simulink model "final_version_control_2026_03_26"  (R2024b)
settings: Solver=FixedStepAuto  StartTime=0.0  StopTime=sim  FixedStep=0.01  RelTol=1e-3  EnableMultiTasking=on
undefined symbols (not defined in the file or in its folder): array, Discrete, K, qbreak, Time
libraries: simulink x71, arduinolib x30, dspswit3 x13, arduinosensorlib x2, ctrlSharedLib x2
(part 3 of 4)

== system final_version_control_2026_03_26/Subsystem3/Right Motor Velocity/Subsystem/Subsystem2 ==
  Enable : Inport
  Velocity : Inport  Port=2
  Mux1 : Mux  Inputs=5
  Subsystem : Subsystem
  Subsystem2 : Subsystem
  Enter_motor_mode : Outport
  Velocity_value : Outport  Port=2
  wires:
  Subsystem2/3(Out3) -> Mux1/3
  Subsystem2/2(Out2) -> Mux1/2
  Subsystem2/4(Out4) -> Mux1/4
  Subsystem2/1(Out1) -> Mux1/1
  Subsystem/1(Out1) -> Velocity_value/1
  Mux1/1 -> Enter_motor_mode/1
  Enable/1 -> Mux1/5
  Velocity/1 -> Subsystem/1(In1)

== system final_version_control_2026_03_26/Subsystem1/Left Motor Velocity1/Motor Actual Position Receive/CHINESE CORRECTION/Subsystem ==
  In1 : Inport
  Enable : EnablePort
  Memory : Memory
  Sum : Sum  Inputs=|++
  Out1 : Outport
  wires:
  In1/1 -> Sum/1
  Sum/1 -> Out1/1, Memory/1
  Memory/1 -> Sum/2

== system final_version_control_2026_03_26/Subsystem1/Left Motor Velocity1/Motor Actual Position Receive/Unpack2/Subsystem ==
  In1 : Inport
  In2 : Inport  Port=2
  In3 : Inport  Port=3
  In4 : Inport  Port=4
  In5 : Inport  Port=5
  Bitwise AND : simulink/Logic and Bit Operations/Bitwise Operator  logicop=AND  UseBitMask=on  BitMask=bin2dec('0000000000001111')  BitMaskRealWorld=Stored Integer
  Bitwise OR : simulink/Logic and Bit Operations/Bitwise Operator  logicop=OR  UseBitMask=off  NumInputPorts=2  BitMask=bin2dec('11011001')  BitMaskRealWorld=Stored Integer
  Bitwise OR1 : simulink/Logic and Bit Operations/Bitwise Operator  logicop=OR  UseBitMask=off  NumInputPorts=2  BitMask=bin2dec('11011001')  BitMaskRealWorld=Stored Integer
  Bitwise OR2 : simulink/Logic and Bit Operations/Bitwise Operator  logicop=OR  UseBitMask=off  NumInputPorts=2  BitMask=bin2dec('11011001')  BitMaskRealWorld=Stored Integer
  Constant : Constant  Value=8  OutDataTypeStr=uint16
  Constant1 : Constant  Value=4  OutDataTypeStr=uint16
  Constant2 : Constant  Value=4  OutDataTypeStr=uint16
  Constant4 : Constant  Value=8  OutDataTypeStr=uint16
  Shift Arithmetic1 : ArithShift  BitShiftNumberSource=Input port  BitShiftNumber=8  BitShiftDirection=Left
  Shift Arithmetic2 : ArithShift  BitShiftNumberSource=Input port  BitShiftNumber=8  BitShiftDirection=Left
  Shift Arithmetic3 : ArithShift  BitShiftNumberSource=Input port  BitShiftNumber=8  BitShiftDirection=Right
  Shift Arithmetic4 : ArithShift  BitShiftNumberSource=Input port  BitShiftNumber=8  BitShiftDirection=Left
  Out1 : Outport
  Out2 : Outport  Port=2
  Out3 : Outport  Port=3
  wires:
  Bitwise AND/1 -> Shift Arithmetic4/1
  In5/1 -> Bitwise OR2/1
  Shift Arithmetic1/1 -> Bitwise OR1/1
  In1/1 -> Shift Arithmetic1/1
  Shift Arithmetic2/1 -> Bitwise OR/1
  Shift Arithmetic3/1 -> Bitwise OR/2
  Shift Arithmetic4/1 -> Bitwise OR2/2
  In2/1 -> Bitwise OR1/2
  Bitwise OR1/1 -> Out1/1
  Bitwise OR2/1 -> Out3/1
  In3/1 -> Shift Arithmetic2/1
  Constant4/1 -> Shift Arithmetic4/2
  Constant2/1 -> Shift Arithmetic3/2
  Constant1/1 -> Shift Arithmetic2/2
  Constant/1 -> Shift Arithmetic1/2
  Bitwise OR/1 -> Out2/1
  In4/1 -> Shift Arithmetic3/1, Bitwise AND/1

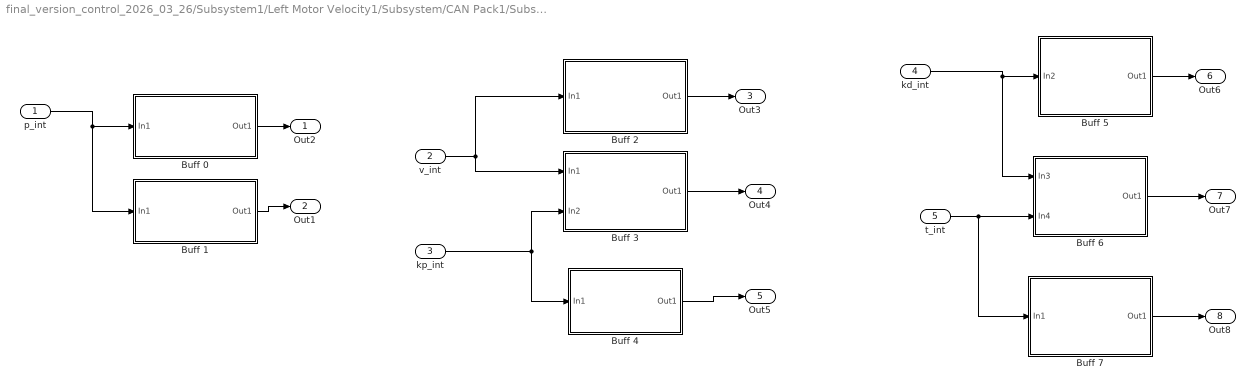
== system final_version_control_2026_03_26/Subsystem1/Left Motor Velocity1/Subsystem/CAN Pack1/Subsystem ==
  p_int : Inport
  v_int : Inport  Port=2
  kp_int : Inport  Port=3
  kd_int : Inport  Port=4
  t_int : Inport  Port=5
  Buff 0 : Subsystem
  Buff 1 : Subsystem
  Buff 2 : Subsystem
  Buff 3 : Subsystem
  Buff 4 : Subsystem
  Buff 5 : Subsystem
  Buff 6 : Subsystem
  Buff 7 : Subsystem
  Out2 : Outport
  Out1 : Outport  Port=2
  Out3 : Outport  Port=3
  Out4 : Outport  Port=4
  Out5 : Outport  Port=5
  Out6 : Outport  Port=6
  Out7 : Outport  Port=7
  Out8 : Outport  Port=8
  wires:
  Buff 5/1(Out1) -> Out6/1
  Buff 7/1(Out1) -> Out8/1
  Buff 6/1(Out1) -> Out7/1
  Buff 0/1(Out1) -> Out2/1
  Buff 1/1(Out1) -> Out1/1
  Buff 2/1(Out1) -> Out3/1
  Buff 4/1(Out1) -> Out5/1
  Buff 3/1(Out1) -> Out4/1
  p_int/1 -> Buff 0/1(In1), Buff 1/1(In1)
  v_int/1 -> Buff 3/1(In1), Buff 2/1(In1)
  kd_int/1 -> Buff 6/1(In3), Buff 5/1(In2)
  kp_int/1 -> Buff 3/2(In2), Buff 4/1(In1)
  t_int/1 -> Buff 7/1(In1), Buff 6/2(In4)

== system final_version_control_2026_03_26/Subsystem1/Left Motor Velocity1/Subsystem/Subsystem2/Subsystem ==
  In1 : Inport
  Kd : Constant  OutDataTypeStr=single
  Kp : Constant  Value=0  OutDataTypeStr=single
  Mux2 : Mux  Inputs=5
  Position Command : Constant  Value=0  VectorParams1D=off  OutDataTypeStr=single
  Saturation : Saturate  UpperLimit=12.5  LowerLimit=-12.5
  Saturation1 : Saturate  UpperLimit=41.87  LowerLimit=-41.87
  Saturation2 : Saturate  UpperLimit=500  LowerLimit=0
  Saturation3 : Saturate  UpperLimit=5  LowerLimit=0
  Saturation4 : Saturate  UpperLimit=9  LowerLimit=-9
  Torque : Constant  Value=0  OutDataTypeStr=single
  Out1 : Outport
  wires:
  Saturation/1 -> Mux2/1
  Kp/1 -> Saturation2/1
  In1/1 -> Saturation1/1
  Position Command/1 -> Saturation/1
  Saturation1/1 -> Mux2/2
  Kd/1 -> Saturation3/1
  Saturation4/1 -> Mux2/5
  Torque/1 -> Saturation4/1
  Saturation2/1 -> Mux2/3
  Saturation3/1 -> Mux2/4
  Mux2/1 -> Out1/1

== system final_version_control_2026_03_26/Subsystem1/Left Motor Velocity1/Subsystem/Subsystem2/Subsystem2 ==
  Kd1 : Constant  Value=5  OutDataTypeStr=single
  Kp1 : Constant  Value=500  OutDataTypeStr=single
  Position Command1 : Constant  Value=12.5  VectorParams1D=off  OutDataTypeStr=single
  Velocity Command1 : Constant  Value=45  OutDataTypeStr=single
  Out1 : Outport
  Out2 : Outport  Port=2
  Out3 : Outport  Port=3
  Out4 : Outport  Port=4
  wires:
  Kd1/1 -> Out4/1
  Position Command1/1 -> Out1/1
  Velocity Command1/1 -> Out2/1
  Kp1/1 -> Out3/1

== system final_version_control_2026_03_26/Subsystem1/Right Motor Velocity1/Motor Actual Position Receive/CHINESE CORRECTION/Subsystem ==
  In1 : Inport
  Enable : EnablePort
  Memory : Memory
  Sum : Sum  Inputs=|++
  Out1 : Outport
  wires:
  In1/1 -> Sum/1
  Sum/1 -> Out1/1, Memory/1
  Memory/1 -> Sum/2

== system final_version_control_2026_03_26/Subsystem1/Right Motor Velocity1/Motor Actual Position Receive/Unpack2/Subsystem ==
  In1 : Inport
  In2 : Inport  Port=2
  In3 : Inport  Port=3
  In4 : Inport  Port=4
  In5 : Inport  Port=5
  Bitwise AND : simulink/Logic and Bit Operations/Bitwise Operator  logicop=AND  UseBitMask=on  BitMask=bin2dec('0000000000001111')  BitMaskRealWorld=Stored Integer
  Bitwise OR : simulink/Logic and Bit Operations/Bitwise Operator  logicop=OR  UseBitMask=off  NumInputPorts=2  BitMask=bin2dec('11011001')  BitMaskRealWorld=Stored Integer
  Bitwise OR1 : simulink/Logic and Bit Operations/Bitwise Operator  logicop=OR  UseBitMask=off  NumInputPorts=2  BitMask=bin2dec('11011001')  BitMaskRealWorld=Stored Integer
  Bitwise OR2 : simulink/Logic and Bit Operations/Bitwise Operator  logicop=OR  UseBitMask=off  NumInputPorts=2  BitMask=bin2dec('11011001')  BitMaskRealWorld=Stored Integer
  Constant : Constant  Value=8  OutDataTypeStr=uint16
  Constant1 : Constant  Value=4  OutDataTypeStr=uint16
  Constant2 : Constant  Value=4  OutDataTypeStr=uint16
  Constant4 : Constant  Value=8  OutDataTypeStr=uint16
  Shift Arithmetic1 : ArithShift  BitShiftNumberSource=Input port  BitShiftNumber=8  BitShiftDirection=Left
  Shift Arithmetic2 : ArithShift  BitShiftNumberSource=Input port  BitShiftNumber=8  BitShiftDirection=Left
  Shift Arithmetic3 : ArithShift  BitShiftNumberSource=Input port  BitShiftNumber=8  BitShiftDirection=Right
  Shift Arithmetic4 : ArithShift  BitShiftNumberSource=Input port  BitShiftNumber=8  BitShiftDirection=Left
  Out1 : Outport
  Out2 : Outport  Port=2
  Out3 : Outport  Port=3
  wires:
  Bitwise AND/1 -> Shift Arithmetic4/1
  In5/1 -> Bitwise OR2/1
  Shift Arithmetic1/1 -> Bitwise OR1/1
  In1/1 -> Shift Arithmetic1/1
  Shift Arithmetic2/1 -> Bitwise OR/1
  Shift Arithmetic3/1 -> Bitwise OR/2
  Shift Arithmetic4/1 -> Bitwise OR2/2
  In2/1 -> Bitwise OR1/2
  Bitwise OR1/1 -> Out1/1
  Bitwise OR2/1 -> Out3/1
  In3/1 -> Shift Arithmetic2/1
  Constant4/1 -> Shift Arithmetic4/2
  Constant2/1 -> Shift Arithmetic3/2
  Constant1/1 -> Shift Arithmetic2/2
  Constant/1 -> Shift Arithmetic1/2
  Bitwise OR/1 -> Out2/1
  In4/1 -> Shift Arithmetic3/1, Bitwise AND/1

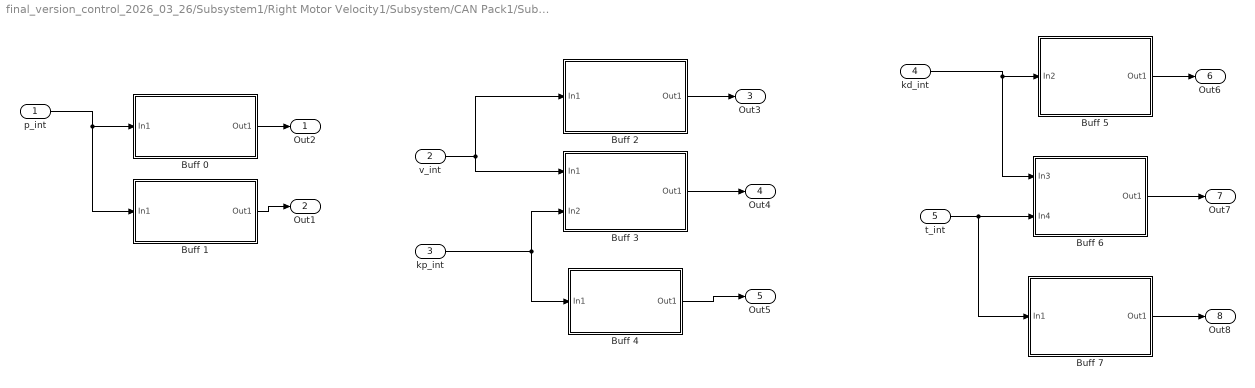
== system final_version_control_2026_03_26/Subsystem1/Right Motor Velocity1/Subsystem/CAN Pack1/Subsystem ==
  p_int : Inport
  v_int : Inport  Port=2
  kp_int : Inport  Port=3
  kd_int : Inport  Port=4
  t_int : Inport  Port=5
  Buff 0 : Subsystem
  Buff 1 : Subsystem
  Buff 2 : Subsystem
  Buff 3 : Subsystem
  Buff 4 : Subsystem
  Buff 5 : Subsystem
  Buff 6 : Subsystem
  Buff 7 : Subsystem
  Out2 : Outport
  Out1 : Outport  Port=2
  Out3 : Outport  Port=3
  Out4 : Outport  Port=4
  Out5 : Outport  Port=5
  Out6 : Outport  Port=6
  Out7 : Outport  Port=7
  Out8 : Outport  Port=8
  wires:
  Buff 5/1(Out1) -> Out6/1
  Buff 7/1(Out1) -> Out8/1
  Buff 6/1(Out1) -> Out7/1
  Buff 0/1(Out1) -> Out2/1
  Buff 1/1(Out1) -> Out1/1
  Buff 2/1(Out1) -> Out3/1
  Buff 4/1(Out1) -> Out5/1
  Buff 3/1(Out1) -> Out4/1
  p_int/1 -> Buff 0/1(In1), Buff 1/1(In1)
  v_int/1 -> Buff 3/1(In1), Buff 2/1(In1)
  kd_int/1 -> Buff 6/1(In3), Buff 5/1(In2)
  kp_int/1 -> Buff 3/2(In2), Buff 4/1(In1)
  t_int/1 -> Buff 7/1(In1), Buff 6/2(In4)

== system final_version_control_2026_03_26/Subsystem1/Right Motor Velocity1/Subsystem/Subsystem2/Subsystem ==
  In1 : Inport
  Kd : Constant  OutDataTypeStr=single
  Kp : Constant  Value=0  OutDataTypeStr=single
  Mux2 : Mux  Inputs=5
  Position Command : Constant  Value=0  VectorParams1D=off  OutDataTypeStr=single
  Saturation : Saturate  UpperLimit=12.5  LowerLimit=-12.5
  Saturation1 : Saturate  UpperLimit=41.87  LowerLimit=-41.87
  Saturation2 : Saturate  UpperLimit=500  LowerLimit=0
  Saturation3 : Saturate  UpperLimit=5  LowerLimit=0
  Saturation4 : Saturate  UpperLimit=9  LowerLimit=-9
  Torque : Constant  Value=0  OutDataTypeStr=single
  Out1 : Outport
  wires:
  Saturation/1 -> Mux2/1
  Kp/1 -> Saturation2/1
  In1/1 -> Saturation1/1
  Position Command/1 -> Saturation/1
  Saturation1/1 -> Mux2/2
  Kd/1 -> Saturation3/1
  Saturation4/1 -> Mux2/5
  Torque/1 -> Saturation4/1
  Saturation2/1 -> Mux2/3
  Saturation3/1 -> Mux2/4
  Mux2/1 -> Out1/1

== system final_version_control_2026_03_26/Subsystem1/Right Motor Velocity1/Subsystem/Subsystem2/Subsystem2 ==
  Kd1 : Constant  Value=5  OutDataTypeStr=single
  Kp1 : Constant  Value=500  OutDataTypeStr=single
  Position Command1 : Constant  Value=12.5  VectorParams1D=off  OutDataTypeStr=single
  Velocity Command1 : Constant  Value=45  OutDataTypeStr=single
  Out1 : Outport
  Out2 : Outport  Port=2
  Out3 : Outport  Port=3
  Out4 : Outport  Port=4
  wires:
  Kd1/1 -> Out4/1
  Position Command1/1 -> Out1/1
  Velocity Command1/1 -> Out2/1
  Kp1/1 -> Out3/1

== system final_version_control_2026_03_26/Subsystem3/Left Motor Velocity/Motor Actual Position Receive/CHINESE CORRECTION/Subsystem ==
  In1 : Inport
  Enable : EnablePort
  Memory : Memory
  Sum : Sum  Inputs=|++
  Out1 : Outport
  wires:
  In1/1 -> Sum/1
  Sum/1 -> Out1/1, Memory/1
  Memory/1 -> Sum/2

== system final_version_control_2026_03_26/Subsystem3/Left Motor Velocity/Motor Actual Position Receive/Unpack2/Subsystem ==
  In1 : Inport
  In2 : Inport  Port=2
  In3 : Inport  Port=3
  In4 : Inport  Port=4
  In5 : Inport  Port=5
  Bitwise AND : simulink/Logic and Bit Operations/Bitwise Operator  logicop=AND  UseBitMask=on  BitMask=bin2dec('0000000000001111')  BitMaskRealWorld=Stored Integer
  Bitwise OR : simulink/Logic and Bit Operations/Bitwise Operator  logicop=OR  UseBitMask=off  NumInputPorts=2  BitMask=bin2dec('11011001')  BitMaskRealWorld=Stored Integer
  Bitwise OR1 : simulink/Logic and Bit Operations/Bitwise Operator  logicop=OR  UseBitMask=off  NumInputPorts=2  BitMask=bin2dec('11011001')  BitMaskRealWorld=Stored Integer
  Bitwise OR2 : simulink/Logic and Bit Operations/Bitwise Operator  logicop=OR  UseBitMask=off  NumInputPorts=2  BitMask=bin2dec('11011001')  BitMaskRealWorld=Stored Integer
  Constant : Constant  Value=8  OutDataTypeStr=uint16
  Constant1 : Constant  Value=4  OutDataTypeStr=uint16
  Constant2 : Constant  Value=4  OutDataTypeStr=uint16
  Constant4 : Constant  Value=8  OutDataTypeStr=uint16
  Shift Arithmetic1 : ArithShift  BitShiftNumberSource=Input port  BitShiftNumber=8  BitShiftDirection=Left
  Shift Arithmetic2 : ArithShift  BitShiftNumberSource=Input port  BitShiftNumber=8  BitShiftDirection=Left
  Shift Arithmetic3 : ArithShift  BitShiftNumberSource=Input port  BitShiftNumber=8  BitShiftDirection=Right
  Shift Arithmetic4 : ArithShift  BitShiftNumberSource=Input port  BitShiftNumber=8  BitShiftDirection=Left
  Out1 : Outport
  Out2 : Outport  Port=2
  Out3 : Outport  Port=3
  wires:
  Bitwise AND/1 -> Shift Arithmetic4/1
  In5/1 -> Bitwise OR2/1
  Shift Arithmetic1/1 -> Bitwise OR1/1
  In1/1 -> Shift Arithmetic1/1
  Shift Arithmetic2/1 -> Bitwise OR/1
  Shift Arithmetic3/1 -> Bitwise OR/2
  Shift Arithmetic4/1 -> Bitwise OR2/2
  In2/1 -> Bitwise OR1/2
  Bitwise OR1/1 -> Out1/1
  Bitwise OR2/1 -> Out3/1
  In3/1 -> Shift Arithmetic2/1
  Constant4/1 -> Shift Arithmetic4/2
  Constant2/1 -> Shift Arithmetic3/2
  Constant1/1 -> Shift Arithmetic2/2
  Constant/1 -> Shift Arithmetic1/2
  Bitwise OR/1 -> Out2/1
  In4/1 -> Shift Arithmetic3/1, Bitwise AND/1

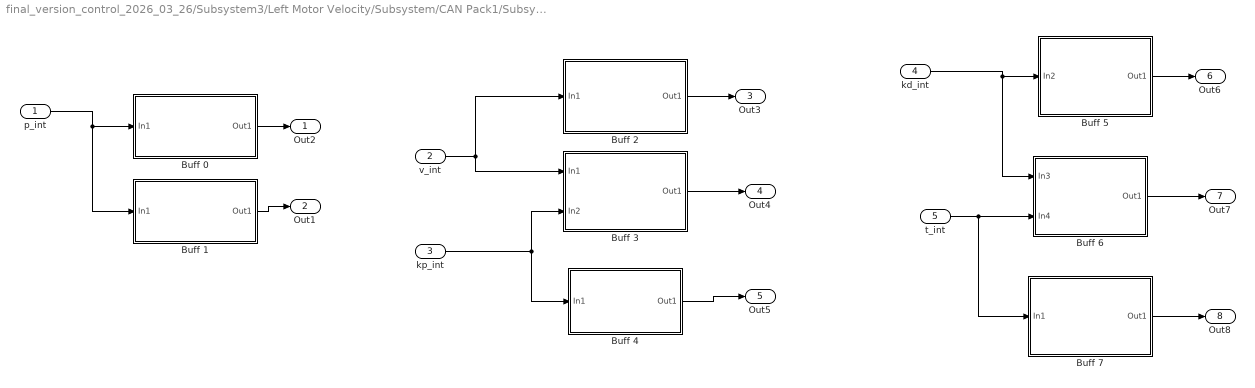
== system final_version_control_2026_03_26/Subsystem3/Left Motor Velocity/Subsystem/CAN Pack1/Subsystem ==
  p_int : Inport
  v_int : Inport  Port=2
  kp_int : Inport  Port=3
  kd_int : Inport  Port=4
  t_int : Inport  Port=5
  Buff 0 : Subsystem
  Buff 1 : Subsystem
  Buff 2 : Subsystem
  Buff 3 : Subsystem
  Buff 4 : Subsystem
  Buff 5 : Subsystem
  Buff 6 : Subsystem
  Buff 7 : Subsystem
  Out2 : Outport
  Out1 : Outport  Port=2
  Out3 : Outport  Port=3
  Out4 : Outport  Port=4
  Out5 : Outport  Port=5
  Out6 : Outport  Port=6
  Out7 : Outport  Port=7
  Out8 : Outport  Port=8
  wires:
  Buff 5/1(Out1) -> Out6/1
  Buff 7/1(Out1) -> Out8/1
  Buff 6/1(Out1) -> Out7/1
  Buff 0/1(Out1) -> Out2/1
  Buff 1/1(Out1) -> Out1/1
  Buff 2/1(Out1) -> Out3/1
  Buff 4/1(Out1) -> Out5/1
  Buff 3/1(Out1) -> Out4/1
  p_int/1 -> Buff 0/1(In1), Buff 1/1(In1)
  v_int/1 -> Buff 3/1(In1), Buff 2/1(In1)
  kd_int/1 -> Buff 6/1(In3), Buff 5/1(In2)
  kp_int/1 -> Buff 3/2(In2), Buff 4/1(In1)
  t_int/1 -> Buff 7/1(In1), Buff 6/2(In4)

== system final_version_control_2026_03_26/Subsystem3/Left Motor Velocity/Subsystem/Subsystem2/Subsystem ==
  In1 : Inport
  Kd : Constant  OutDataTypeStr=single
  Kp : Constant  Value=0  OutDataTypeStr=single
  Mux2 : Mux  Inputs=5
  Position Command : Constant  Value=0  VectorParams1D=off  OutDataTypeStr=single
  Saturation : Saturate  UpperLimit=12.5  LowerLimit=-12.5
  Saturation1 : Saturate  UpperLimit=41.87  LowerLimit=-41.87
  Saturation2 : Saturate  UpperLimit=500  LowerLimit=0
  Saturation3 : Saturate  UpperLimit=5  LowerLimit=0
  Saturation4 : Saturate  UpperLimit=9  LowerLimit=-9
  Torque : Constant  Value=0  OutDataTypeStr=single
  Out1 : Outport
  wires:
  Saturation/1 -> Mux2/1
  Kp/1 -> Saturation2/1
  In1/1 -> Saturation1/1
  Position Command/1 -> Saturation/1
  Saturation1/1 -> Mux2/2
  Kd/1 -> Saturation3/1
  Saturation4/1 -> Mux2/5
  Torque/1 -> Saturation4/1
  Saturation2/1 -> Mux2/3
  Saturation3/1 -> Mux2/4
  Mux2/1 -> Out1/1

== system final_version_control_2026_03_26/Subsystem3/Left Motor Velocity/Subsystem/Subsystem2/Subsystem2 ==
  Kd1 : Constant  Value=5  OutDataTypeStr=single
  Kp1 : Constant  Value=500  OutDataTypeStr=single
  Position Command1 : Constant  Value=12.5  VectorParams1D=off  OutDataTypeStr=single
  Velocity Command1 : Constant  Value=45  OutDataTypeStr=single
  Out1 : Outport
  Out2 : Outport  Port=2
  Out3 : Outport  Port=3
  Out4 : Outport  Port=4
  wires:
  Kd1/1 -> Out4/1
  Position Command1/1 -> Out1/1
  Velocity Command1/1 -> Out2/1
  Kp1/1 -> Out3/1

== system final_version_control_2026_03_26/Subsystem3/Right Motor Velocity/Motor Actual Position Receive/CHINESE CORRECTION/Subsystem ==
  In1 : Inport
  Enable : EnablePort
  Memory : Memory
  Sum : Sum  Inputs=|++
  Out1 : Outport
  wires:
  In1/1 -> Sum/1
  Sum/1 -> Out1/1, Memory/1
  Memory/1 -> Sum/2

== system final_version_control_2026_03_26/Subsystem3/Right Motor Velocity/Motor Actual Position Receive/Unpack2/Subsystem ==
  In1 : Inport
  In2 : Inport  Port=2
  In3 : Inport  Port=3
  In4 : Inport  Port=4
  In5 : Inport  Port=5
  Bitwise AND : simulink/Logic and Bit Operations/Bitwise Operator  logicop=AND  UseBitMask=on  BitMask=bin2dec('0000000000001111')  BitMaskRealWorld=Stored Integer
  Bitwise OR : simulink/Logic and Bit Operations/Bitwise Operator  logicop=OR  UseBitMask=off  NumInputPorts=2  BitMask=bin2dec('11011001')  BitMaskRealWorld=Stored Integer
  Bitwise OR1 : simulink/Logic and Bit Operations/Bitwise Operator  logicop=OR  UseBitMask=off  NumInputPorts=2  BitMask=bin2dec('11011001')  BitMaskRealWorld=Stored Integer
  Bitwise OR2 : simulink/Logic and Bit Operations/Bitwise Operator  logicop=OR  UseBitMask=off  NumInputPorts=2  BitMask=bin2dec('11011001')  BitMaskRealWorld=Stored Integer
  Constant : Constant  Value=8  OutDataTypeStr=uint16
  Constant1 : Constant  Value=4  OutDataTypeStr=uint16
  Constant2 : Constant  Value=4  OutDataTypeStr=uint16
  Constant4 : Constant  Value=8  OutDataTypeStr=uint16
  Shift Arithmetic1 : ArithShift  BitShiftNumberSource=Input port  BitShiftNumber=8  BitShiftDirection=Left
  Shift Arithmetic2 : ArithShift  BitShiftNumberSource=Input port  BitShiftNumber=8  BitShiftDirection=Left
  Shift Arithmetic3 : ArithShift  BitShiftNumberSource=Input port  BitShiftNumber=8  BitShiftDirection=Right
  Shift Arithmetic4 : ArithShift  BitShiftNumberSource=Input port  BitShiftNumber=8  BitShiftDirection=Left
  Out1 : Outport
  Out2 : Outport  Port=2
  Out3 : Outport  Port=3
  wires:
  Bitwise AND/1 -> Shift Arithmetic4/1
  In5/1 -> Bitwise OR2/1
  Shift Arithmetic1/1 -> Bitwise OR1/1
  In1/1 -> Shift Arithmetic1/1
  Shift Arithmetic2/1 -> Bitwise OR/1
  Shift Arithmetic3/1 -> Bitwise OR/2
  Shift Arithmetic4/1 -> Bitwise OR2/2
  In2/1 -> Bitwise OR1/2
  Bitwise OR1/1 -> Out1/1
  Bitwise OR2/1 -> Out3/1
  In3/1 -> Shift Arithmetic2/1
  Constant4/1 -> Shift Arithmetic4/2
  Constant2/1 -> Shift Arithmetic3/2
  Constant1/1 -> Shift Arithmetic2/2
  Constant/1 -> Shift Arithmetic1/2
  Bitwise OR/1 -> Out2/1
  In4/1 -> Shift Arithmetic3/1, Bitwise AND/1

== system final_version_control_2026_03_26/Subsystem3/Right Motor Velocity/Subsystem/CAN Pack1/Subsystem ==
  p_int : Inport
  v_int : Inport  Port=2
  kp_int : Inport  Port=3
  kd_int : Inport  Port=4
  t_int : Inport  Port=5
  Buff 0 : Subsystem
  Buff 1 : Subsystem
  Buff 2 : Subsystem
  Buff 3 : Subsystem
  Buff 4 : Subsystem
  Buff 5 : Subsystem
  Buff 6 : Subsystem
  Buff 7 : Subsystem
  Out2 : Outport
  Out1 : Outport  Port=2
  Out3 : Outport  Port=3
  Out4 : Outport  Port=4
  Out5 : Outport  Port=5
  Out6 : Outport  Port=6
  Out7 : Outport  Port=7
  Out8 : Outport  Port=8
  wires:
  Buff 5/1(Out1) -> Out6/1
  Buff 7/1(Out1) -> Out8/1
  Buff 6/1(Out1) -> Out7/1
  Buff 0/1(Out1) -> Out2/1
  Buff 1/1(Out1) -> Out1/1
  Buff 2/1(Out1) -> Out3/1
  Buff 4/1(Out1) -> Out5/1
  Buff 3/1(Out1) -> Out4/1
  p_int/1 -> Buff 0/1(In1), Buff 1/1(In1)
  v_int/1 -> Buff 3/1(In1), Buff 2/1(In1)
  kd_int/1 -> Buff 6/1(In3), Buff 5/1(In2)
  kp_int/1 -> Buff 3/2(In2), Buff 4/1(In1)
  t_int/1 -> Buff 7/1(In1), Buff 6/2(In4)

== system final_version_control_2026_03_26/Subsystem3/Right Motor Velocity/Subsystem/Subsystem2/Subsystem ==
  In1 : Inport
  Kd : Constant  OutDataTypeStr=single
  Kp : Constant  Value=0  OutDataTypeStr=single
  Mux2 : Mux  Inputs=5
  Position Command : Constant  Value=0  VectorParams1D=off  OutDataTypeStr=single
  Saturation : Saturate  UpperLimit=12.5  LowerLimit=-12.5
  Saturation1 : Saturate  UpperLimit=41.87  LowerLimit=-41.87
  Saturation2 : Saturate  UpperLimit=500  LowerLimit=0
  Saturation3 : Saturate  UpperLimit=5  LowerLimit=0
  Saturation4 : Saturate  UpperLimit=9  LowerLimit=-9
  Torque : Constant  Value=0  OutDataTypeStr=single
  Out1 : Outport
  wires:
  Saturation/1 -> Mux2/1
  Kp/1 -> Saturation2/1
  In1/1 -> Saturation1/1
  Position Command/1 -> Saturation/1
  Saturation1/1 -> Mux2/2
  Kd/1 -> Saturation3/1
  Saturation4/1 -> Mux2/5
  Torque/1 -> Saturation4/1
  Saturation2/1 -> Mux2/3
  Saturation3/1 -> Mux2/4
  Mux2/1 -> Out1/1

== system final_version_control_2026_03_26/Subsystem3/Right Motor Velocity/Subsystem/Subsystem2/Subsystem2 ==
  Kd1 : Constant  Value=5  OutDataTypeStr=single
  Kp1 : Constant  Value=500  OutDataTypeStr=single
  Position Command1 : Constant  Value=12.5  VectorParams1D=off  OutDataTypeStr=single
  Velocity Command1 : Constant  Value=45  OutDataTypeStr=single
  Out1 : Outport
  Out2 : Outport  Port=2
  Out3 : Outport  Port=3
  Out4 : Outport  Port=4
  wires:
  Kd1/1 -> Out4/1
  Position Command1/1 -> Out1/1
  Velocity Command1/1 -> Out2/1
  Kp1/1 -> Out3/1

== system final_version_control_2026_03_26/Subsystem1/Left Motor Velocity1/Subsystem/CAN Pack1/Subsystem/Buff 0 ==
  In1 : Inport
  Constant1 : Constant  Value=8  OutDataTypeStr=uint16
  Data Type Conversion : DataTypeConversion  OutDataTypeStr=uint8  SaturateOnIntegerOverflow=off  RndMeth=Floor
  Shift Arithmetic2 : ArithShift  BitShiftNumberSource=Input port  BitShiftNumber=8  BitShiftDirection=Right
  Out1 : Outport
  wires:
  In1/1 -> Shift Arithmetic2/1
  Shift Arithmetic2/1 -> Data Type Conversion/1
  Data Type Conversion/1 -> Out1/1
  Constant1/1 -> Shift Arithmetic2/2

== system final_version_control_2026_03_26/Subsystem1/Left Motor Velocity1/Subsystem/CAN Pack1/Subsystem/Buff 1 ==
  In1 : Inport
  Bitwise AND : simulink/Logic and Bit Operations/Bitwise Operator  logicop=AND  UseBitMask=on  BitMask=bin2dec('0000000011111111')  BitMaskRealWorld=Stored Integer
  Data Type Conversion1 : DataTypeConversion  OutDataTypeStr=uint8  SaturateOnIntegerOverflow=off  RndMeth=Floor
  Out1 : Outport
  wires:
  Bitwise AND/1 -> Data Type Conversion1/1
  Data Type Conversion1/1 -> Out1/1
  In1/1 -> Bitwise AND/1

== system final_version_control_2026_03_26/Subsystem1/Left Motor Velocity1/Subsystem/CAN Pack1/Subsystem/Buff 2 ==
  In1 : Inport
  Constant2 : Constant  Value=4  OutDataTypeStr=uint16
  Data Type Conversion2 : DataTypeConversion  OutDataTypeStr=uint8  SaturateOnIntegerOverflow=off  RndMeth=Floor
  Shift Arithmetic1 : ArithShift  BitShiftNumberSource=Input port  BitShiftNumber=8  BitShiftDirection=Right
  Out1 : Outport
  wires:
  Shift Arithmetic1/1 -> Data Type Conversion2/1
  Data Type Conversion2/1 -> Out1/1
  In1/1 -> Shift Arithmetic1/1
  Constant2/1 -> Shift Arithmetic1/2

== system final_version_control_2026_03_26/Subsystem1/Left Motor Velocity1/Subsystem/CAN Pack1/Subsystem/Buff 3 ==
  In1 : Inport
  In2 : Inport  Port=2
  Bitwise AND1 : simulink/Logic and Bit Operations/Bitwise Operator  logicop=AND  UseBitMask=on  BitMask=bin2dec('000000001111')  BitMaskRealWorld=Stored Integer
  Bitwise OR1 : simulink/Logic and Bit Operations/Bitwise Operator  logicop=OR  UseBitMask=off  NumInputPorts=2  BitMask=bin2dec('11011001')  BitMaskRealWorld=Stored Integer
  Constant1 : Constant  Value=8  OutDataTypeStr=uint16
  Constant2 : Constant  Value=4  OutDataTypeStr=uint16
  Data Type Conversion3 : DataTypeConversion  OutDataTypeStr=uint8  SaturateOnIntegerOverflow=off  RndMeth=Floor
  Shift Arithmetic3 : ArithShift  BitShiftNumberSource=Input port  BitShiftNumber=8  BitShiftDirection=Left
  Shift Arithmetic4 : ArithShift  BitShiftNumberSource=Input port  BitShiftNumber=8  BitShiftDirection=Right
  Out1 : Outport
  wires:
  Shift Arithmetic3/1 -> Bitwise OR1/1
  In1/1 -> Bitwise AND1/1
  Constant1/1 -> Shift Arithmetic4/2
  Bitwise AND1/1 -> Shift Arithmetic3/1
  Shift Arithmetic4/1 -> Bitwise OR1/2
  In2/1 -> Shift Arithmetic4/1
  Bitwise OR1/1 -> Data Type Conversion3/1
  Data Type Conversion3/1 -> Out1/1
  Constant2/1 -> Shift Arithmetic3/2

== system final_version_control_2026_03_26/Subsystem1/Left Motor Velocity1/Subsystem/CAN Pack1/Subsystem/Buff 4 ==
  In1 : Inport
  Bitwise AND3 : simulink/Logic and Bit Operations/Bitwise Operator  logicop=AND  UseBitMask=on  BitMask=bin2dec('000011111111')  BitMaskRealWorld=Stored Integer
  Data Type Conversion4 : DataTypeConversion  OutDataTypeStr=uint8  SaturateOnIntegerOverflow=off  RndMeth=Floor
  Out1 : Outport
  wires:
  Data Type Conversion4/1 -> Out1/1
  Bitwise AND3/1 -> Data Type Conversion4/1
  In1/1 -> Bitwise AND3/1

== system final_version_control_2026_03_26/Subsystem1/Left Motor Velocity1/Subsystem/CAN Pack1/Subsystem/Buff 5 ==
  In2 : Inport
  Constant2 : Constant  Value=4  OutDataTypeStr=uint16
  Data Type Conversion5 : DataTypeConversion  OutDataTypeStr=uint8  SaturateOnIntegerOverflow=off  RndMeth=Floor
  Shift Arithmetic5 : ArithShift  BitShiftNumberSource=Input port  BitShiftNumber=8  BitShiftDirection=Right
  Out1 : Outport
  wires:
  In2/1 -> Shift Arithmetic5/1
  Shift Arithmetic5/1 -> Data Type Conversion5/1
  Data Type Conversion5/1 -> Out1/1
  Constant2/1 -> Shift Arithmetic5/2

== system final_version_control_2026_03_26/Subsystem1/Left Motor Velocity1/Subsystem/CAN Pack1/Subsystem/Buff 6 ==
  In3 : Inport
  In4 : Inport  Port=2
  Bitwise AND2 : simulink/Logic and Bit Operations/Bitwise Operator  logicop=AND  UseBitMask=on  BitMask=bin2dec('000000001111')  BitMaskRealWorld=Stored Integer
  Bitwise OR2 : simulink/Logic and Bit Operations/Bitwise Operator  logicop=OR  UseBitMask=off  NumInputPorts=2  BitMask=bin2dec('11011001')  BitMaskRealWorld=Stored Integer
  Constant1 : Constant  Value=8  OutDataTypeStr=uint16
  Constant2 : Constant  Value=4  OutDataTypeStr=uint16
  Data Type Conversion6 : DataTypeConversion  OutDataTypeStr=uint8  SaturateOnIntegerOverflow=off  RndMeth=Floor
  Shift Arithmetic6 : ArithShift  BitShiftNumberSource=Input port  BitShiftNumber=8  BitShiftDirection=Left
  Shift Arithmetic7 : ArithShift  BitShiftNumberSource=Input port  BitShiftNumber=8  BitShiftDirection=Right
  Out1 : Outport
  wires:
  In4/1 -> Shift Arithmetic7/1
  Shift Arithmetic7/1 -> Bitwise OR2/2
  Shift Arithmetic6/1 -> Bitwise OR2/1
  Bitwise OR2/1 -> Data Type Conversion6/1
  In3/1 -> Bitwise AND2/1
  Bitwise AND2/1 -> Shift Arithmetic6/1
  Data Type Conversion6/1 -> Out1/1
  Constant2/1 -> Shift Arithmetic6/2
  Constant1/1 -> Shift Arithmetic7/2

== system final_version_control_2026_03_26/Subsystem1/Left Motor Velocity1/Subsystem/CAN Pack1/Subsystem/Buff 7 ==
  In1 : Inport
  Bitwise AND4 : simulink/Logic and Bit Operations/Bitwise Operator  logicop=AND  UseBitMask=on  BitMask=bin2dec('000011111111')  BitMaskRealWorld=Stored Integer
  Data Type Conversion7 : DataTypeConversion  OutDataTypeStr=uint8  SaturateOnIntegerOverflow=off  RndMeth=Floor
  Out1 : Outport
  wires:
  Bitwise AND4/1 -> Data Type Conversion7/1
  Data Type Conversion7/1 -> Out1/1
  In1/1 -> Bitwise AND4/1

== system final_version_control_2026_03_26/Subsystem1/Right Motor Velocity1/Subsystem/CAN Pack1/Subsystem/Buff 0 ==
  In1 : Inport
  Constant1 : Constant  Value=8  OutDataTypeStr=uint16
  Data Type Conversion : DataTypeConversion  OutDataTypeStr=uint8  SaturateOnIntegerOverflow=off  RndMeth=Floor
  Shift Arithmetic2 : ArithShift  BitShiftNumberSource=Input port  BitShiftNumber=8  BitShiftDirection=Right
  Out1 : Outport
  wires:
  In1/1 -> Shift Arithmetic2/1
  Shift Arithmetic2/1 -> Data Type Conversion/1
  Data Type Conversion/1 -> Out1/1
  Constant1/1 -> Shift Arithmetic2/2

== system final_version_control_2026_03_26/Subsystem1/Right Motor Velocity1/Subsystem/CAN Pack1/Subsystem/Buff 1 ==
  In1 : Inport
  Bitwise AND : simulink/Logic and Bit Operations/Bitwise Operator  logicop=AND  UseBitMask=on  BitMask=bin2dec('0000000011111111')  BitMaskRealWorld=Stored Integer
  Data Type Conversion1 : DataTypeConversion  OutDataTypeStr=uint8  SaturateOnIntegerOverflow=off  RndMeth=Floor
  Out1 : Outport
  wires:
  Bitwise AND/1 -> Data Type Conversion1/1
  Data Type Conversion1/1 -> Out1/1
  In1/1 -> Bitwise AND/1

== system final_version_control_2026_03_26/Subsystem1/Right Motor Velocity1/Subsystem/CAN Pack1/Subsystem/Buff 2 ==
  In1 : Inport
  Constant2 : Constant  Value=4  OutDataTypeStr=uint16
  Data Type Conversion2 : DataTypeConversion  OutDataTypeStr=uint8  SaturateOnIntegerOverflow=off  RndMeth=Floor
  Shift Arithmetic1 : ArithShift  BitShiftNumberSource=Input port  BitShiftNumber=8  BitShiftDirection=Right
  Out1 : Outport
  wires:
  Shift Arithmetic1/1 -> Data Type Conversion2/1
  Data Type Conversion2/1 -> Out1/1
  In1/1 -> Shift Arithmetic1/1
  Constant2/1 -> Shift Arithmetic1/2

== system final_version_control_2026_03_26/Subsystem1/Right Motor Velocity1/Subsystem/CAN Pack1/Subsystem/Buff 3 ==
  In1 : Inport
  In2 : Inport  Port=2
  Bitwise AND1 : simulink/Logic and Bit Operations/Bitwise Operator  logicop=AND  UseBitMask=on  BitMask=bin2dec('000000001111')  BitMaskRealWorld=Stored Integer
  Bitwise OR1 : simulink/Logic and Bit Operations/Bitwise Operator  logicop=OR  UseBitMask=off  NumInputPorts=2  BitMask=bin2dec('11011001')  BitMaskRealWorld=Stored Integer
  Constant1 : Constant  Value=8  OutDataTypeStr=uint16
  Constant2 : Constant  Value=4  OutDataTypeStr=uint16
  Data Type Conversion3 : DataTypeConversion  OutDataTypeStr=uint8  SaturateOnIntegerOverflow=off  RndMeth=Floor
  Shift Arithmetic3 : ArithShift  BitShiftNumberSource=Input port  BitShiftNumber=8  BitShiftDirection=Left
  Shift Arithmetic4 : ArithShift  BitShiftNumberSource=Input port  BitShiftNumber=8  BitShiftDirection=Right
  Out1 : Outport
  wires:
  Shift Arithmetic3/1 -> Bitwise OR1/1
  In1/1 -> Bitwise AND1/1
  Constant1/1 -> Shift Arithmetic4/2
  Bitwise AND1/1 -> Shift Arithmetic3/1
  Shift Arithmetic4/1 -> Bitwise OR1/2
  In2/1 -> Shift Arithmetic4/1
  Bitwise OR1/1 -> Data Type Conversion3/1
  Data Type Conversion3/1 -> Out1/1
  Constant2/1 -> Shift Arithmetic3/2

== system final_version_control_2026_03_26/Subsystem1/Right Motor Velocity1/Subsystem/CAN Pack1/Subsystem/Buff 4 ==
  In1 : Inport
  Bitwise AND3 : simulink/Logic and Bit Operations/Bitwise Operator  logicop=AND  UseBitMask=on  BitMask=bin2dec('000011111111')  BitMaskRealWorld=Stored Integer
  Data Type Conversion4 : DataTypeConversion  OutDataTypeStr=uint8  SaturateOnIntegerOverflow=off  RndMeth=Floor
  Out1 : Outport
  wires:
  Data Type Conversion4/1 -> Out1/1
  Bitwise AND3/1 -> Data Type Conversion4/1
  In1/1 -> Bitwise AND3/1

== system final_version_control_2026_03_26/Subsystem1/Right Motor Velocity1/Subsystem/CAN Pack1/Subsystem/Buff 5 ==
  In2 : Inport
  Constant2 : Constant  Value=4  OutDataTypeStr=uint16
  Data Type Conversion5 : DataTypeConversion  OutDataTypeStr=uint8  SaturateOnIntegerOverflow=off  RndMeth=Floor
  Shift Arithmetic5 : ArithShift  BitShiftNumberSource=Input port  BitShiftNumber=8  BitShiftDirection=Right
  Out1 : Outport
  wires:
  In2/1 -> Shift Arithmetic5/1
  Shift Arithmetic5/1 -> Data Type Conversion5/1
  Data Type Conversion5/1 -> Out1/1
  Constant2/1 -> Shift Arithmetic5/2

== system final_version_control_2026_03_26/Subsystem1/Right Motor Velocity1/Subsystem/CAN Pack1/Subsystem/Buff 6 ==
  In3 : Inport
  In4 : Inport  Port=2
  Bitwise AND2 : simulink/Logic and Bit Operations/Bitwise Operator  logicop=AND  UseBitMask=on  BitMask=bin2dec('000000001111')  BitMaskRealWorld=Stored Integer
  Bitwise OR2 : simulink/Logic and Bit Operations/Bitwise Operator  logicop=OR  UseBitMask=off  NumInputPorts=2  BitMask=bin2dec('11011001')  BitMaskRealWorld=Stored Integer
  Constant1 : Constant  Value=8  OutDataTypeStr=uint16
  Constant2 : Constant  Value=4  OutDataTypeStr=uint16
  Data Type Conversion6 : DataTypeConversion  OutDataTypeStr=uint8  SaturateOnIntegerOverflow=off  RndMeth=Floor
  Shift Arithmetic6 : ArithShift  BitShiftNumberSource=Input port  BitShiftNumber=8  BitShiftDirection=Left
  Shift Arithmetic7 : ArithShift  BitShiftNumberSource=Input port  BitShiftNumber=8  BitShiftDirection=Right
  Out1 : Outport
  wires:
  In4/1 -> Shift Arithmetic7/1
  Shift Arithmetic7/1 -> Bitwise OR2/2
  Shift Arithmetic6/1 -> Bitwise OR2/1
  Bitwise OR2/1 -> Data Type Conversion6/1
  In3/1 -> Bitwise AND2/1
  Bitwise AND2/1 -> Shift Arithmetic6/1
  Data Type Conversion6/1 -> Out1/1
  Constant2/1 -> Shift Arithmetic6/2
  Constant1/1 -> Shift Arithmetic7/2

== system final_version_control_2026_03_26/Subsystem1/Right Motor Velocity1/Subsystem/CAN Pack1/Subsystem/Buff 7 ==
  In1 : Inport
  Bitwise AND4 : simulink/Logic and Bit Operations/Bitwise Operator  logicop=AND  UseBitMask=on  BitMask=bin2dec('000011111111')  BitMaskRealWorld=Stored Integer
  Data Type Conversion7 : DataTypeConversion  OutDataTypeStr=uint8  SaturateOnIntegerOverflow=off  RndMeth=Floor
  Out1 : Outport
  wires:
  Bitwise AND4/1 -> Data Type Conversion7/1
  Data Type Conversion7/1 -> Out1/1
  In1/1 -> Bitwise AND4/1

== system final_version_control_2026_03_26/Subsystem3/Left Motor Velocity/Subsystem/CAN Pack1/Subsystem/Buff 0 ==
  In1 : Inport
  Constant1 : Constant  Value=8  OutDataTypeStr=uint16
  Data Type Conversion : DataTypeConversion  OutDataTypeStr=uint8  SaturateOnIntegerOverflow=off  RndMeth=Floor
  Shift Arithmetic2 : ArithShift  BitShiftNumberSource=Input port  BitShiftNumber=8  BitShiftDirection=Right
  Out1 : Outport
  wires:
  In1/1 -> Shift Arithmetic2/1
  Shift Arithmetic2/1 -> Data Type Conversion/1
  Data Type Conversion/1 -> Out1/1
  Constant1/1 -> Shift Arithmetic2/2

== system final_version_control_2026_03_26/Subsystem3/Left Motor Velocity/Subsystem/CAN Pack1/Subsystem/Buff 1 ==
  In1 : Inport
  Bitwise AND : simulink/Logic and Bit Operations/Bitwise Operator  logicop=AND  UseBitMask=on  BitMask=bin2dec('0000000011111111')  BitMaskRealWorld=Stored Integer
  Data Type Conversion1 : DataTypeConversion  OutDataTypeStr=uint8  SaturateOnIntegerOverflow=off  RndMeth=Floor
  Out1 : Outport
  wires:
  Bitwise AND/1 -> Data Type Conversion1/1
  Data Type Conversion1/1 -> Out1/1
  In1/1 -> Bitwise AND/1

== system final_version_control_2026_03_26/Subsystem3/Left Motor Velocity/Subsystem/CAN Pack1/Subsystem/Buff 2 ==
  In1 : Inport
  Constant2 : Constant  Value=4  OutDataTypeStr=uint16
  Data Type Conversion2 : DataTypeConversion  OutDataTypeStr=uint8  SaturateOnIntegerOverflow=off  RndMeth=Floor
  Shift Arithmetic1 : ArithShift  BitShiftNumberSource=Input port  BitShiftNumber=8  BitShiftDirection=Right
  Out1 : Outport
  wires:
  Shift Arithmetic1/1 -> Data Type Conversion2/1
  Data Type Conversion2/1 -> Out1/1
  In1/1 -> Shift Arithmetic1/1
  Constant2/1 -> Shift Arithmetic1/2

== system final_version_control_2026_03_26/Subsystem3/Left Motor Velocity/Subsystem/CAN Pack1/Subsystem/Buff 3 ==
  In1 : Inport
  In2 : Inport  Port=2
  Bitwise AND1 : simulink/Logic and Bit Operations/Bitwise Operator  logicop=AND  UseBitMask=on  BitMask=bin2dec('000000001111')  BitMaskRealWorld=Stored Integer
  Bitwise OR1 : simulink/Logic and Bit Operations/Bitwise Operator  logicop=OR  UseBitMask=off  NumInputPorts=2  BitMask=bin2dec('11011001')  BitMaskRealWorld=Stored Integer
  Constant1 : Constant  Value=8  OutDataTypeStr=uint16
  Constant2 : Constant  Value=4  OutDataTypeStr=uint16
  Data Type Conversion3 : DataTypeConversion  OutDataTypeStr=uint8  SaturateOnIntegerOverflow=off  RndMeth=Floor
  Shift Arithmetic3 : ArithShift  BitShiftNumberSource=Input port  BitShiftNumber=8  BitShiftDirection=Left
  Shift Arithmetic4 : ArithShift  BitShiftNumberSource=Input port  BitShiftNumber=8  BitShiftDirection=Right
  Out1 : Outport
  wires:
  Shift Arithmetic3/1 -> Bitwise OR1/1
  In1/1 -> Bitwise AND1/1
  Constant1/1 -> Shift Arithmetic4/2
  Bitwise AND1/1 -> Shift Arithmetic3/1
  Shift Arithmetic4/1 -> Bitwise OR1/2
  In2/1 -> Shift Arithmetic4/1
  Bitwise OR1/1 -> Data Type Conversion3/1
  Data Type Conversion3/1 -> Out1/1
  Constant2/1 -> Shift Arithmetic3/2

== system final_version_control_2026_03_26/Subsystem3/Left Motor Velocity/Subsystem/CAN Pack1/Subsystem/Buff 4 ==
  In1 : Inport
  Bitwise AND3 : simulink/Logic and Bit Operations/Bitwise Operator  logicop=AND  UseBitMask=on  BitMask=bin2dec('000011111111')  BitMaskRealWorld=Stored Integer
  Data Type Conversion4 : DataTypeConversion  OutDataTypeStr=uint8  SaturateOnIntegerOverflow=off  RndMeth=Floor
  Out1 : Outport
  wires:
  Data Type Conversion4/1 -> Out1/1
  Bitwise AND3/1 -> Data Type Conversion4/1
  In1/1 -> Bitwise AND3/1

== system final_version_control_2026_03_26/Subsystem3/Left Motor Velocity/Subsystem/CAN Pack1/Subsystem/Buff 5 ==
  In2 : Inport
  Constant2 : Constant  Value=4  OutDataTypeStr=uint16
  Data Type Conversion5 : DataTypeConversion  OutDataTypeStr=uint8  SaturateOnIntegerOverflow=off  RndMeth=Floor
  Shift Arithmetic5 : ArithShift  BitShiftNumberSource=Input port  BitShiftNumber=8  BitShiftDirection=Right
  Out1 : Outport
  wires:
  In2/1 -> Shift Arithmetic5/1
  Shift Arithmetic5/1 -> Data Type Conversion5/1
  Data Type Conversion5/1 -> Out1/1
  Constant2/1 -> Shift Arithmetic5/2

== system final_version_control_2026_03_26/Subsystem3/Left Motor Velocity/Subsystem/CAN Pack1/Subsystem/Buff 6 ==
  In3 : Inport
  In4 : Inport  Port=2
  Bitwise AND2 : simulink/Logic and Bit Operations/Bitwise Operator  logicop=AND  UseBitMask=on  BitMask=bin2dec('000000001111')  BitMaskRealWorld=Stored Integer
  Bitwise OR2 : simulink/Logic and Bit Operations/Bitwise Operator  logicop=OR  UseBitMask=off  NumInputPorts=2  BitMask=bin2dec('11011001')  BitMaskRealWorld=Stored Integer
  Constant1 : Constant  Value=8  OutDataTypeStr=uint16
  Constant2 : Constant  Value=4  OutDataTypeStr=uint16
  Data Type Conversion6 : DataTypeConversion  OutDataTypeStr=uint8  SaturateOnIntegerOverflow=off  RndMeth=Floor
  Shift Arithmetic6 : ArithShift  BitShiftNumberSource=Input port  BitShiftNumber=8  BitShiftDirection=Left
  Shift Arithmetic7 : ArithShift  BitShiftNumberSource=Input port  BitShiftNumber=8  BitShiftDirection=Right
  Out1 : Outport
  wires:
  In4/1 -> Shift Arithmetic7/1
  Shift Arithmetic7/1 -> Bitwise OR2/2
  Shift Arithmetic6/1 -> Bitwise OR2/1
  Bitwise OR2/1 -> Data Type Conversion6/1
  In3/1 -> Bitwise AND2/1
  Bitwise AND2/1 -> Shift Arithmetic6/1
  Data Type Conversion6/1 -> Out1/1
  Constant2/1 -> Shift Arithmetic6/2
  Constant1/1 -> Shift Arithmetic7/2

== system final_version_control_2026_03_26/Subsystem3/Left Motor Velocity/Subsystem/CAN Pack1/Subsystem/Buff 7 ==
  In1 : Inport
  Bitwise AND4 : simulink/Logic and Bit Operations/Bitwise Operator  logicop=AND  UseBitMask=on  BitMask=bin2dec('000011111111')  BitMaskRealWorld=Stored Integer
  Data Type Conversion7 : DataTypeConversion  OutDataTypeStr=uint8  SaturateOnIntegerOverflow=off  RndMeth=Floor
  Out1 : Outport
  wires:
  Bitwise AND4/1 -> Data Type Conversion7/1
  Data Type Conversion7/1 -> Out1/1
  In1/1 -> Bitwise AND4/1

== system final_version_control_2026_03_26/Subsystem3/Right Motor Velocity/Subsystem/CAN Pack1/Subsystem/Buff 0 ==
  In1 : Inport
  Constant1 : Constant  Value=8  OutDataTypeStr=uint16
  Data Type Conversion : DataTypeConversion  OutDataTypeStr=uint8  SaturateOnIntegerOverflow=off  RndMeth=Floor
  Shift Arithmetic2 : ArithShift  BitShiftNumberSource=Input port  BitShiftNumber=8  BitShiftDirection=Right
  Out1 : Outport
  wires:
  In1/1 -> Shift Arithmetic2/1
  Shift Arithmetic2/1 -> Data Type Conversion/1
  Data Type Conversion/1 -> Out1/1
  Constant1/1 -> Shift Arithmetic2/2

== system final_version_control_2026_03_26/Subsystem3/Right Motor Velocity/Subsystem/CAN Pack1/Subsystem/Buff 1 ==
  In1 : Inport
  Bitwise AND : simulink/Logic and Bit Operations/Bitwise Operator  logicop=AND  UseBitMask=on  BitMask=bin2dec('0000000011111111')  BitMaskRealWorld=Stored Integer
  Data Type Conversion1 : DataTypeConversion  OutDataTypeStr=uint8  SaturateOnIntegerOverflow=off  RndMeth=Floor
  Out1 : Outport
  wires:
  Bitwise AND/1 -> Data Type Conversion1/1
  Data Type Conversion1/1 -> Out1/1
  In1/1 -> Bitwise AND/1

== system final_version_control_2026_03_26/Subsystem3/Right Motor Velocity/Subsystem/CAN Pack1/Subsystem/Buff 2 ==
  In1 : Inport
  Constant2 : Constant  Value=4  OutDataTypeStr=uint16
  Data Type Conversion2 : DataTypeConversion  OutDataTypeStr=uint8  SaturateOnIntegerOverflow=off  RndMeth=Floor
  Shift Arithmetic1 : ArithShift  BitShiftNumberSource=Input port  BitShiftNumber=8  BitShiftDirection=Right
  Out1 : Outport
  wires:
  Shift Arithmetic1/1 -> Data Type Conversion2/1
  Data Type Conversion2/1 -> Out1/1
  In1/1 -> Shift Arithmetic1/1
  Constant2/1 -> Shift Arithmetic1/2

== system final_version_control_2026_03_26/Subsystem3/Right Motor Velocity/Subsystem/CAN Pack1/Subsystem/Buff 3 ==
  In1 : Inport
  In2 : Inport  Port=2
  Bitwise AND1 : simulink/Logic and Bit Operations/Bitwise Operator  logicop=AND  UseBitMask=on  BitMask=bin2dec('000000001111')  BitMaskRealWorld=Stored Integer
  Bitwise OR1 : simulink/Logic and Bit Operations/Bitwise Operator  logicop=OR  UseBitMask=off  NumInputPorts=2  BitMask=bin2dec('11011001')  BitMaskRealWorld=Stored Integer
  Constant1 : Constant  Value=8  OutDataTypeStr=uint16
  Constant2 : Constant  Value=4  OutDataTypeStr=uint16
  Data Type Conversion3 : DataTypeConversion  OutDataTypeStr=uint8  SaturateOnIntegerOverflow=off  RndMeth=Floor
  Shift Arithmetic3 : ArithShift  BitShiftNumberSource=Input port  BitShiftNumber=8  BitShiftDirection=Left
  Shift Arithmetic4 : ArithShift  BitShiftNumberSource=Input port  BitShiftNumber=8  BitShiftDirection=Right
  Out1 : Outport
  wires:
  Shift Arithmetic3/1 -> Bitwise OR1/1
  In1/1 -> Bitwise AND1/1
  Constant1/1 -> Shift Arithmetic4/2
  Bitwise AND1/1 -> Shift Arithmetic3/1
  Shift Arithmetic4/1 -> Bitwise OR1/2
  In2/1 -> Shift Arithmetic4/1
  Bitwise OR1/1 -> Data Type Conversion3/1
  Data Type Conversion3/1 -> Out1/1
  Constant2/1 -> Shift Arithmetic3/2

== system final_version_control_2026_03_26/Subsystem3/Right Motor Velocity/Subsystem/CAN Pack1/Subsystem/Buff 4 ==
  In1 : Inport
  Bitwise AND3 : simulink/Logic and Bit Operations/Bitwise Operator  logicop=AND  UseBitMask=on  BitMask=bin2dec('000011111111')  BitMaskRealWorld=Stored Integer
  Data Type Conversion4 : DataTypeConversion  OutDataTypeStr=uint8  SaturateOnIntegerOverflow=off  RndMeth=Floor
  Out1 : Outport
  wires:
  Data Type Conversion4/1 -> Out1/1
  Bitwise AND3/1 -> Data Type Conversion4/1
  In1/1 -> Bitwise AND3/1

== system final_version_control_2026_03_26/Subsystem3/Right Motor Velocity/Subsystem/CAN Pack1/Subsystem/Buff 5 ==
  In2 : Inport
  Constant2 : Constant  Value=4  OutDataTypeStr=uint16
  Data Type Conversion5 : DataTypeConversion  OutDataTypeStr=uint8  SaturateOnIntegerOverflow=off  RndMeth=Floor
  Shift Arithmetic5 : ArithShift  BitShiftNumberSource=Input port  BitShiftNumber=8  BitShiftDirection=Right
  Out1 : Outport
  wires:
  In2/1 -> Shift Arithmetic5/1
  Shift Arithmetic5/1 -> Data Type Conversion5/1
  Data Type Conversion5/1 -> Out1/1
  Constant2/1 -> Shift Arithmetic5/2

== system final_version_control_2026_03_26/Subsystem3/Right Motor Velocity/Subsystem/CAN Pack1/Subsystem/Buff 6 ==
  In3 : Inport
  In4 : Inport  Port=2
  Bitwise AND2 : simulink/Logic and Bit Operations/Bitwise Operator  logicop=AND  UseBitMask=on  BitMask=bin2dec('000000001111')  BitMaskRealWorld=Stored Integer
  Bitwise OR2 : simulink/Logic and Bit Operations/Bitwise Operator  logicop=OR  UseBitMask=off  NumInputPorts=2  BitMask=bin2dec('11011001')  BitMaskRealWorld=Stored Integer
  Constant1 : Constant  Value=8  OutDataTypeStr=uint16
  Constant2 : Constant  Value=4  OutDataTypeStr=uint16
  Data Type Conversion6 : DataTypeConversion  OutDataTypeStr=uint8  SaturateOnIntegerOverflow=off  RndMeth=Floor
  Shift Arithmetic6 : ArithShift  BitShiftNumberSource=Input port  BitShiftNumber=8  BitShiftDirection=Left
  Shift Arithmetic7 : ArithShift  BitShiftNumberSource=Input port  BitShiftNumber=8  BitShiftDirection=Right
  Out1 : Outport
  wires:
  In4/1 -> Shift Arithmetic7/1
  Shift Arithmetic7/1 -> Bitwise OR2/2
  Shift Arithmetic6/1 -> Bitwise OR2/1
  Bitwise OR2/1 -> Data Type Conversion6/1
  In3/1 -> Bitwise AND2/1
  Bitwise AND2/1 -> Shift Arithmetic6/1
  Data Type Conversion6/1 -> Out1/1
  Constant2/1 -> Shift Arithmetic6/2
  Constant1/1 -> Shift Arithmetic7/2

== system final_version_control_2026_03_26/Subsystem3/Right Motor Velocity/Subsystem/CAN Pack1/Subsystem/Buff 7 ==
  In1 : Inport
  Bitwise AND4 : simulink/Logic and Bit Operations/Bitwise Operator  logicop=AND  UseBitMask=on  BitMask=bin2dec('000011111111')  BitMaskRealWorld=Stored Integer
  Data Type Conversion7 : DataTypeConversion  OutDataTypeStr=uint8  SaturateOnIntegerOverflow=off  RndMeth=Floor
  Out1 : Outport
  wires:
  Bitwise AND4/1 -> Data Type Conversion7/1
  Data Type Conversion7/1 -> Out1/1
  In1/1 -> Bitwise AND4/1

== stateflow chart final_version_control_2026_03_26/RIGHT LEG/Subsystem/Chart1 ==
  state LG
    gain=amplitude;
    sigmoid_power = sig_power;
    scale_LM = Scale;
  state DS
    gain=amplitude-0.5;
    sigmoid_power = sig_power+100;
    scale_LM = Scale - 0.5;
  state AS
    gain=amplitude+2;
    sigmoid_power = sig_power+100;
    scale_LM = Scale - 0.6;
  (default) -> LG
  DS -> LG [order 1] : [class==0]
  LG -> DS [order 2] : [class==2]
  LG -> AS [order 1] : [class==1]
  AS -> LG [order 2] : [class==0]
  AS -> DS [order 1] : [class==2]
  DS -> AS [order 2] : [class==1]
  data: scale_LM output; class input; gain output; amplitude input; sigmoid_power output; sig_power input; scale_LM input; Scale input

== matlab function final_version_control_2026_03_26/IMUs/SOGI + FLL (IN PHASE + QUADRATURE COMPONENT ESTIMATION)1/MATLAB Function1 ==
  settings: updateMethod=DISCRETE
function [theta, theta_quad] = SOGI_FLL( ...
    x, Ts, ...
    f_min, f_max, ...     % cadence bounds (walking/running range)
    k_sogi, k_fll, ...            % FLL adaptation speed (sensor/noise dependent)
    E_lo, E_hi)           % lock thresholds (amplitude/noise dependent)


% SOGI-FLL:
%   SOGI = Second-Order Generalized Integrator (generates in-phase + quadrature)
%   FLL  = Frequency-Locked Loop (adapts internal frequency to cadence changes)
%
% INPUTS:
%   x       : drift-removed joint angle [rad] (recommended: x = theta_raw - slowLPF(theta_raw))
%   walking : boolean gate (true when moving; false when standing)
%   Ts      : sample time [s]
%
%   f_min,f_max : [Hz] plausible cadence bounds (include running if needed)
%   k_fll       : FLL adaptation gain (higher=faster, more sensitive to noise)
%   E_lo,E_hi   : energy thresholds for confidence/lock (depends on amplitude & noise)
%
% OUTPUTS:
%   theta       : in-phase filtered signal
%   theta_quad  : quadrature signal

%% -------- Fixed “rarely changed” parameters (keep inside) --------

walking = 1.0; %walking detected

fc_f_smooth = 0.30;
% Tune only if internal frequency becomes jittery or too laggy:
%   - decrease to 0.2 for smoother (more lag)
%   - increase to 0.5 for faster (more jitter)

fc_lock = 0.50;
% Tune only if lock flickers or reacts too slowly:
%   - decrease (0.3) to reduce flicker
%   - increase (0.8–1.0) for faster start/stop response

f_init = 1.4;              % [Hz] initial guess (walking/running general default)
% Tune only if you want faster lock at startup:
%   - set near typical cadence in your trials (walk ~1–2 Hz, run ~2–3 Hz)

decay_notwalking = 0.999;   % state decay when standing
% Tune only if oscillator rings too long after stopping:
%   - faster decay: 0.995
%   - slower decay: 0.9995

epsSmall = 1e-9;            % numerical safety
% Increase only if you see NaN/Inf in extreme low-motion segments (e.g., 1e-8)

%% -------------------- Persistent states --------------------
persistent va vb w_est f_state lock_state
if isempty(va)
    va = 0; vb = 0;
    w_est = 2*pi*f_init;
    f_state = f_init;
    lock_state = 0;
end

%% -------------------- Precompute smoothing coefficients --------------------
aF    = exp(-2*pi*fc_f_smooth*Ts);
aLock = exp(-2*pi*fc_lock*Ts);

%% -------------------- Frequency bounds in rad/s --------------------
w_min = 2*pi*f_min;
w_max = 2*pi*f_max;

w0 = clamp(w_est, w_min, w_max);

%% ==================== SOGI ====================
if walking
    e = x - va;

    va = va + Ts*( w0*vb + k_sogi*w0*e );
    vb = vb + Ts*( -w0*va );
else
    va = decay_notwalking*va;
    vb = decay_notwalking*vb;
    e  = 0;
end

theta = va;
theta_quad = vb;

%% ==================== Lock/confidence ====================
E = theta*theta + theta_quad*theta_quad;
lock_state = aLock*lock_state + (1-aLock)*E;

lock = clamp((lock_state - E_lo)/(E_hi - E_lo + epsSmall), 0, 1);

%% ==================== FLL ====================
if walking
    mu = (e * theta_quad) / (E + epsSmall);

    w_est = w0 + Ts * (k_fll * w0 * mu) * lock;
    w_est = clamp(w_est, w_min, w_max);

    f_raw = w_est/(2*pi);
    f_state = aF*f_state + (1-aF)*f_raw;

    w_est = 2*pi*clamp(f_state, f_min, f_max);
else
    f_state = 0.995*f_state + 0.005*f_init;
    w_est   = 2*pi*f_state;
end

end

function y = clamp(x, lo, hi)
y = min(max(x, lo), hi);
end
